simulink model "Interferometer_High_gain_Luiz"  (R2019b)
settings: Solver=ode3  StartTime=0.0  StopTime=5  FixedStep=0.00001  RelTol=1e-3
undefined symbols (not defined in the file or in its folder): sgn
libraries: simulink x1
settings Model: Creator=Stinky  LastModifiedBy=Stinky

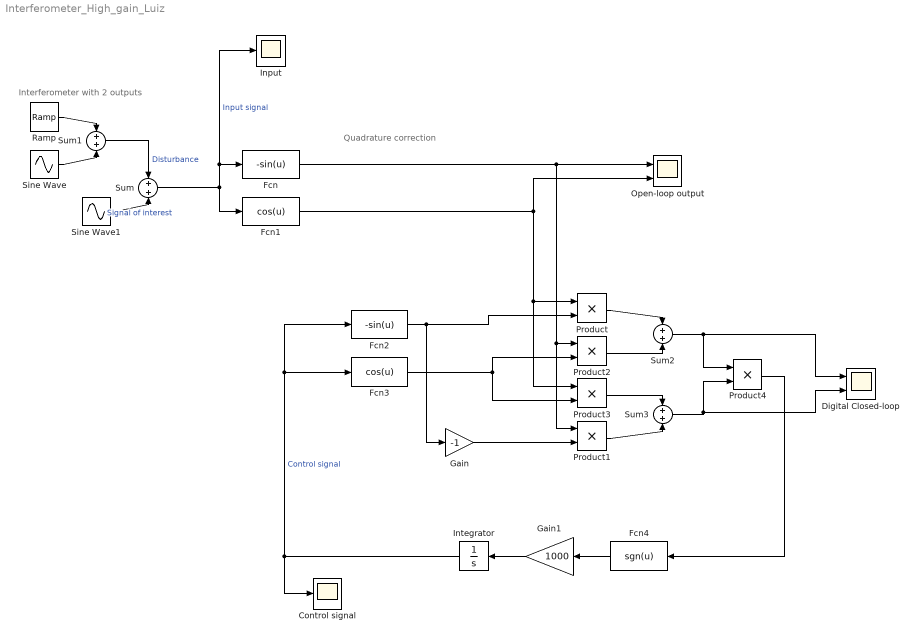
== system Interferometer_High_gain_Luiz ==
  note: Quadrature correction
  note: Interferometer with 2 outputs
  Control signal : Scope
  Digital Closed-loop : Scope  NumInputPorts=2
  Fcn : Fcn  Expr=-sin(u)
  Fcn1 : Fcn  Expr=cos(u)
  Fcn2 : Fcn  Expr=-sin(u)
  Fcn3 : Fcn  Expr=cos(u)
  Fcn4 : Fcn  Expr=sgn(u)
  Gain : Gain  Gain=-1
  Gain1 : Gain  Gain=1000
  Input : Scope
  Integrator : Integrator
  Open-loop output : Scope  NumInputPorts=2
  Product{,1..4} (5 alike) : Product
  Ramp : simulink/Sources/Ramp  slope=0.1  start=0  InitialOutput=0
  Sine Wave : Sin  Frequency=0.1  SampleTime=0
  Sine Wave1 : Sin  Amplitude=5  Frequency=100  SampleTime=0
  Sum{,1..3} (4 alike) : Sum  Inputs=+|+
  wires:
  Sine Wave1/1 -> Sum/2  "Signal of interest"
  Sum/1 -> Input/1, Fcn/1, Fcn1/1  "Input signal"
  Ramp/1 -> Sum1/1
  Sine Wave/1 -> Sum1/2
  Sum1/1 -> Sum/1  "Disturbance"
  Fcn1/1 -> Product3/1, Product/1, Open-loop output/2
  Fcn2/1 -> Gain/1, Product/2
  Fcn/1 -> Open-loop output/1, Product1/1, Product2/1
  Fcn3/1 -> Product3/2, Product2/2
  Gain/1 -> Product1/2
  Product/1 -> Sum2/1
  Product2/1 -> Sum2/2
  Product3/1 -> Sum3/1
  Product1/1 -> Sum3/2
  Sum2/1 -> Digital Closed-loop/1, Product4/1
  Sum3/1 -> Digital Closed-loop/2, Product4/2
  Integrator/1 -> Fcn3/1, Fcn2/1, Control signal/1  "Control signal"
  Gain1/1 -> Integrator/1
  Fcn4/1 -> Gain1/1
  Product4/1 -> Fcn4/1
